simulink model "esdStatsTest"  (R2020b)
settings: Solver=FixedStepDiscrete  StartTime=0.0  StopTime=stopTime  RelTol=1e-3
PostLoadFcn:
  | addpath([fileparts(which(bdroot)) filesep '..' filesep])
  | loadDataSimulinkCallback
InitFcn:
  | simulinkInitEsdStats
StopFcn:
  | simulinkVerifyEsdStats
undefined symbols (not defined in the file or in its folder): params
libraries: dspsrcs4 x1
settings Model: DataTypeOverride=Off  SimulationMode=accelerator  Creator=trevor  LastModifiedBy=trevor
settings DataIOCC: SaveFormat=Array  SaveOutput=off  DSMLogging=off  SaveTime=off  ReturnWorkspaceOutputs=off
settings OptimizationCC: BlockReduction=off  ConditionallyExecuteInputs=off  DefaultParameterBehavior=Inlined
settings DebuggingCC: AlgebraicLoopMsg=error  SingleTaskRateTransMsg=error  SFMachineParentedDataDiag=error
settings HardwareCC: ProdBitPerPointer=32  ProdBitPerSizeT=32  ProdBitPerPtrDiffT=32  ProdLargestAtomicFloat=None  ProdIntDivRoundTo=Undefined  ProdEndianess=Unspecified  ProdWordSize=32  ProdHWDeviceType=ASIC/FPGA->ASIC/FPGA  TargetBitPerLong=64  TargetBitPerPointer=64  TargetBitPerSizeT=64  TargetBitPerPtrDiffT=64  TargetLongLongMode=on  TargetIntDivRoundTo=Zero  TargetEndianess=LittleEndian  TargetWordSize=64  TargetHWDeviceType=Custom Processor->MATLAB Host Computer  ProdEqTarget=off

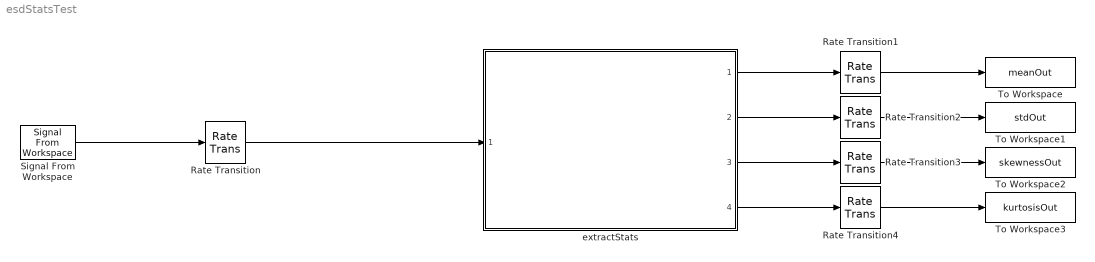
== system esdStatsTest ==
  Rate Transition : RateTransition  Deterministic=off  OutPortSampleTime=params.systemClockPeriod
  Rate Transition{1..4} (4 alike) : RateTransition  OutPortSampleTime=params.samplingPeriod
  Signal From Workspace : dspsrcs4/Signal From Workspace  X=esd  Ts=params.samplingPeriod  nsamps=1  OutputAfterFinalValue=Setting to zero  ignoreOrWarnInputAndFrameLengths=off  OutputFrames=off
  To Workspace : ToWorkspace  VariableName=meanOut  SampleTime=-1
      settings: Save2DSignal=2-D array (concatenate along first dimension)
  To Workspace1 : ToWorkspace  VariableName=stdOut  SampleTime=-1
      settings: Save2DSignal=2-D array (concatenate along first dimension)
  To Workspace2 : ToWorkspace  VariableName=skewnessOut  SampleTime=-1
      settings: Save2DSignal=2-D array (concatenate along first dimension)
  To Workspace3 : ToWorkspace  VariableName=kurtosisOut  SampleTime=-1
      settings: Save2DSignal=2-D array (concatenate along first dimension)
  extractStats : Subsystem  ReferencedSubsystem=extractEsdStats
  wires:
  Signal From Workspace/1 -> Rate Transition/1
  Rate Transition1/1 -> To Workspace/1
  extractStats/1 -> Rate Transition1/1
  Rate Transition/1 -> extractStats/1
  Rate Transition2/1 -> To Workspace1/1
  Rate Transition3/1 -> To Workspace2/1
  Rate Transition4/1 -> To Workspace3/1
  extractStats/4 -> Rate Transition4/1
  extractStats/3 -> Rate Transition3/1
  extractStats/2 -> Rate Transition2/1
